simulink model "ACC_detailed_model2"  (R2018a)
settings: Solver=VariableStepAuto  StartTime=0.0  StopTime=250  FixedStep=1e-3  RelTol=1e-3
InitFcn:
  | Jw = 4.5; % Inertia Kg.m^2
  | r = 0.3; % Radius of Wheel
  | Cf = 0.1; % Viscous coefficient
  | 
  | r=0.3; % Radius of wheel
  |  %Dry Asphalt road%
  | C1 = 1.2801;
  | C2 = 23.99;
  | C3 = 0.52;
  | 
  | M = 1300; % 1500Kg
  | g = 9.81; % m/s2
  | Cr = 0.01;				% coefficient of rolling friction
  | rho = 1.3;				% density of air, kg/m^3
  | Cd = 0.46;% drag coefficient
  | 
  | maxspeed=30;
  | Alarm1=0;  %Initializing the Alarm
  | speed1=0;  %Initializing the speed
  | Default_Spacing_distance = 5; % Default Safe distance between both vehicles
  | THW= 1.5; %Time Headway
  | min_distance = 2; % Minimum Distance
libraries: simulink x5
settings Model: Creator=CHIZOM WORNU  LastModifiedBy=CHIZOM WORNU
settings SolverCC: ConsecutiveZCsStepRelTol=1*128*eps  ZeroCrossControl=EnableAll  ZeroCrossAlgorithm=Adaptive

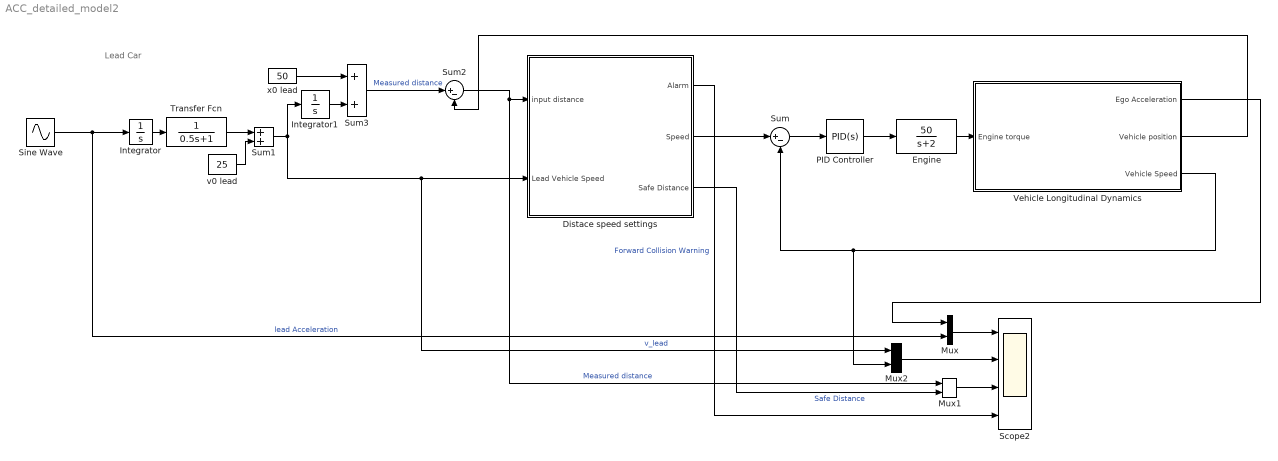
== system ACC_detailed_model2 ==
  note: Lead Car
  Distace speed settings : Subsystem
  Engine : TransferFcn  Numerator=50  Denominator=[1 2]
  Integrator : Integrator
  Integrator1 : Integrator  InitialCondition=10
  Mux : Mux  Inputs=2
  Mux1 : Mux  Inputs=2
  Mux2 : Mux  Inputs=2
  PID Controller : simulink/Continuous/PID Controller  Controller=PID  TimeDomain=Continuous-time  SampleTime=-1  IntegratorMethod=Forward Euler  FilterMethod=Forward Euler  Form=Parallel  UseFilter=on  ControllerParametersSource=internal  P=30.0096454190468  I=4.39323599940394  D=-0.171141386307986  N=175.350019457254  InitialConditionSource=internal  InitialConditionForIntegrator=0  InitialConditionForFilter=0  ExternalReset=none  LimitOutput=off  UpperSaturationLimit=inf  LowerSaturationLimit=-inf  LinearizeAsGain=on  AntiWindupMode=none  Kb=1  TrackingMode=off  Kt=1  PParamMin=[]  PParamMax=[]  IParamMin=[]  IParamMax=[]  DParamMin=[]  DParamMax=[]  NParamMin=[]  NParamMax=[]  KbParamMin=[]  KbParamMax=[]  KtParamMin=[]  KtParamMax=[]  POutMin=[]  POutMax=[]  IOutMin=[]  IOutMax=[]  DOutMin=[]  DOutMax=[]  NOutMin=[]  NOutMax=[]  KbOutMin=[]  KbOutMax=[]  KtOutMin=[]  KtOutMax=[]  IntegratorOutMin=[]  IntegratorOutMax=[]  FilterOutMin=[]  FilterOutMax=[]  SumOutMin=[]  SumOutMax=[]  SumI1OutMin=[]  SumI1OutMax=[]  SumI2OutMin=[]  SumI2OutMax=[]  SumI3OutMin=[]  SumI3OutMax=[]  SumDOutMin=[]  SumDOutMax=[]  SaturationOutMin=[]  SaturationOutMax=[]  IntegratorContinuousStateAttributes=''  IntegratorStateMustResolveToSignalObject=off  IntegratorRTWStateStorageClass=Auto  FilterContinuousStateAttributes=''  FilterStateMustResolveToSignalObject=off  FilterRTWStateStorageClass=Auto  DifferentiatorICPrevScaledInput=0  DifferentiatorOutMin=[]  DifferentiatorOutMax=[]  InitialConditionSetting=State (most efficient)  FilterDiffOutCoefMin=[]  FilterDiffOutCoefMax=[]  SumDenOutMin=[]  SumDenOutMax=[]  SumNumOutMin=[]  SumNumOutMax=[]  ReciprocalOutMin=[]  ReciprocalOutMax=[]  DivideOutMin=[]  DivideOutMax=[]  TunerSelectOption=Transfer Function Based (PID Tuner App)
  Scope2 : Scope  NumInputPorts=4
  Sine Wave : Sin  Amplitude=0.5  Frequency=0.2  SampleTime=0.1
  Sum : Sum  Inputs=|+-
  Sum1 : Sum
  Sum2 : Sum  Inputs=|+-
  Sum3 : Sum
  Transfer Fcn : TransferFcn  Denominator=[0.5 1]
  Vehicle Longitudinal Dynamics : Subsystem
  v0 lead : Constant  Value=25  SampleTime=0.1
  x0 lead : Constant  Value=50  SampleTime=0.1
  wires:
  Mux/1 -> Scope2/1
  Sum/1 -> PID Controller/1
  PID Controller/1 -> Engine/1
  Sum2/1 -> Distace speed settings/1(input distance), Mux1/1  "Measured distance"
  Sum1/1 -> Distace speed settings/2(Lead Vehicle Speed), Mux2/1, Integrator1/1  "v_lead"
  Sine Wave/1 -> Mux/2, Integrator/1  "lead Acceleration"
  Sum3/1 -> Sum2/1  "Measured distance"
  Mux2/1 -> Scope2/2
  Mux1/1 -> Scope2/3
  Integrator1/1 -> Sum3/2
  x0 lead/1 -> Sum3/1
  Integrator/1 -> Transfer Fcn/1
  v0 lead/1 -> Sum1/2
  Transfer Fcn/1 -> Sum1/1
  Engine/1 -> Vehicle Longitudinal Dynamics/1(Engine torque)
  Vehicle Longitudinal Dynamics/1(Ego Acceleration) -> Mux/1
  Distace speed settings/1(Alarm) -> Scope2/4  "Forward Collision Warning"
  Distace speed settings/2(Speed) -> Sum/1
  Distace speed settings/3(Safe Distance) -> Mux1/2  "Safe Distance"
  Vehicle Longitudinal Dynamics/2(Vehicle position) -> Sum2/2
  Vehicle Longitudinal Dynamics/3(Vehicle Speed) -> Sum/2, Mux2/2

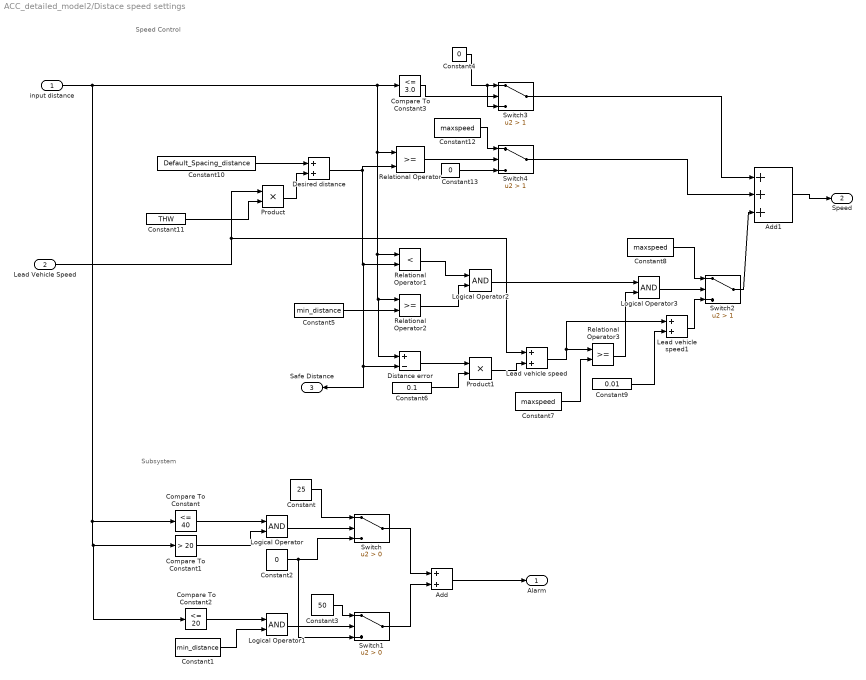
== system ACC_detailed_model2/Distace speed settings ==
  note: Speed Control
  note: Subsystem
  input distance : Inport
  Lead Vehicle Speed : Inport  Port=2
  Add : Sum
  Add1 : Sum  Inputs=3
  Compare To Constant : simulink/Logic and Bit Operations/Compare To Constant  relop=<=  const=40  OutDataTypeStr=boolean
  Compare To Constant1 : simulink/Logic and Bit Operations/Compare To Constant  relop=>  const=20  OutDataTypeStr=boolean
  Compare To Constant2 : simulink/Logic and Bit Operations/Compare To Constant  relop=<=  const=20  OutDataTypeStr=boolean
  Compare To Constant3 : simulink/Logic and Bit Operations/Compare To Constant  relop=<=  const=3.0  OutDataTypeStr=boolean
  Constant : Constant  Value=25
  Constant1 : Constant  Value=min_distance
  Constant10 : Constant  Value=Default_Spacing_distance
  Constant11 : Constant  Value=THW
  Constant12 : Constant  Value=maxspeed
  Constant13 : Constant  Value=0
  Constant2 : Constant  Value=0
  Constant3 : Constant  Value=50
  Constant4 : Constant  Value=0
  Constant5 : Constant  Value=min_distance
  Constant6 : Constant  Value=0.1
  Constant7 : Constant  Value=maxspeed
  Constant8 : Constant  Value=maxspeed
  Constant9 : Constant  Value=0.01
  Desired distance : Sum
  Distance error : Sum  Inputs=+-
  Lead vehicle speed : Sum
  Lead vehicle speed1 : Sum
  Logical Operator{,1..3} (4 alike) : Logic  AllPortsSameDT=off  OutDataTypeStr=boolean
  Product : Product
  Product1 : Product
  Relational Operator : RelationalOperator  OutDataTypeStr=boolean  RndMeth=Simplest
  Relational Operator1 : RelationalOperator  Operator=<  OutDataTypeStr=boolean  RndMeth=Simplest
  Relational Operator2 : RelationalOperator  OutDataTypeStr=boolean  RndMeth=Simplest
  Relational Operator3 : RelationalOperator  OutDataTypeStr=boolean  RndMeth=Simplest
  Switch : Switch  Criteria=u2 > Threshold
  Switch1 : Switch  Criteria=u2 > Threshold
  Switch2 : Switch  Criteria=u2 > Threshold  Threshold=1
  Switch3 : Switch  Criteria=u2 > Threshold  Threshold=1
  Switch4 : Switch  Criteria=u2 > Threshold  Threshold=1
  Alarm : Outport
  Speed : Outport  Port=2
  Safe Distance : Outport  Port=3
  wires:
  Add/1 -> Alarm/1
  Lead vehicle speed/1 -> Lead vehicle speed1/1, Relational Operator3/1
  Add1/1 -> Speed/1
  Desired distance/1 -> Distance error/2, Safe Distance/1, Relational Operator1/2, Relational Operator/2
  Switch/1 -> Add/1
  Constant1/1 -> Logical Operator1/2
  Constant3/1 -> Switch1/1
  Logical Operator1/1 -> Switch1/2
  Compare To Constant/1 -> Logical Operator/1
  Logical Operator/1 -> Switch/2
  Compare To Constant1/1 -> Logical Operator/2
  Constant2/1 -> Switch1/3, Switch/3
  Switch1/1 -> Add/2
  Constant/1 -> Switch/1
  Compare To Constant2/1 -> Logical Operator1/1
  Switch3/1 -> Add1/1
  Constant13/1 -> Switch4/3
  Constant10/1 -> Desired distance/1
  Constant9/1 -> Lead vehicle speed1/2
  Constant4/1 -> Switch3/3, Switch3/1
  Product1/1 -> Lead vehicle speed/2
  Relational Operator1/1 -> Logical Operator2/1
  Constant8/1 -> Switch2/1
  Lead vehicle speed1/1 -> Switch2/3
  Distance error/1 -> Product1/1
  Constant5/1 -> Relational Operator2/2
  Relational Operator/1 -> Switch4/2
  Product/1 -> Desired distance/2
  Constant11/1 -> Product/2
  Constant7/1 -> Relational Operator3/2
  Switch2/1 -> Add1/3
  Constant12/1 -> Switch4/1
  Logical Operator2/1 -> Logical Operator3/1
  Switch4/1 -> Add1/2
  Logical Operator3/1 -> Switch2/2
  Constant6/1 -> Product1/2
  Compare To Constant3/1 -> Switch3/2
  Lead Vehicle Speed/1 -> Product/1, Lead vehicle speed/1
  Relational Operator3/1 -> Logical Operator3/2
  input distance/1 -> Compare To Constant2/1, Compare To Constant1/1, Compare To Constant/1, Compare To Constant3/1, Distance error/1, Relational Operator2/1, Relational Operator1/1, Relational Operator/1
  Relational Operator2/1 -> Logical Operator2/2

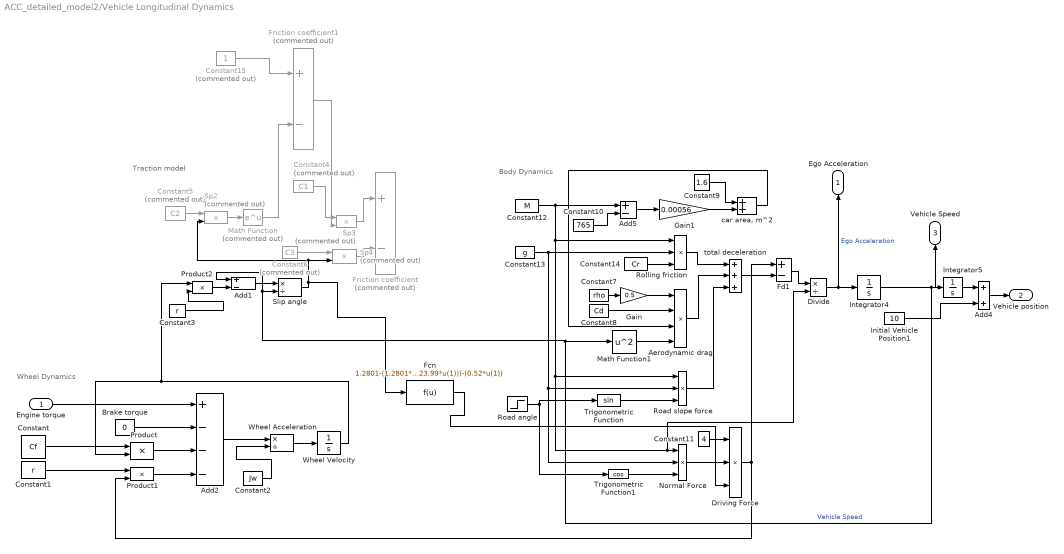
== system ACC_detailed_model2/Vehicle Longitudinal Dynamics ==
  note: Body Dynamics
  note: Traction model
  note: Wheel Dynamics
  Engine torque : Inport
  Add1 : Sum  Inputs=+-
  Add2 : Sum  Inputs=+---
  Add4 : Sum
  Add5 : Sum  Inputs=+-
  Aerodynamic drag : Product  Inputs=4
  Brake torque : Constant  Value=0
  Constant : Constant  Value=Cf
  Constant1 : Constant  Value=r
  Constant10 : Constant  Value=765
  Constant11 : Constant  Value=4
  Constant12 : Constant  Value=M
  Constant13 : Constant  Value=g
  Constant14 : Constant  Value=Cr
  Constant15 : Constant  Commented=on
  Constant2 : Constant  Value=Jw
  Constant3 : Constant  Value=r
  Constant4 : Constant  Commented=on  Value=C1
  Constant5 : Constant  Commented=on  Value=C2
  Constant6 : Constant  Commented=on  Value=C3
  Constant7 : Constant  Value=rho
  Constant8 : Constant  Value=Cd
  Constant9 : Constant  Value=1.6
  Divide : Product  Inputs=*/
  Driving Force : Product  Inputs=3
  Fcn : Fcn  Expr=1.2801-(1.2801*exp(23.99*u(1)))-(0.52*u(1))
  Fd1 : Sum  Inputs=+-
  Friction coefficient : Sum  Commented=on  Inputs=+-
  Friction coefficient1 : Sum  Commented=on  Inputs=+-
  Gain : Gain  Gain=0.5
  Gain1 : Gain  Gain=0.00056
  Initial Vehicle Position1 : Constant  Value=10  SampleTime=0.1
  Integrator4 : Integrator  InitialCondition=1
  Integrator5 : Integrator  InitialCondition=1
  Math Function : Math  Commented=on  SaturateOnIntegerOverflow=on
  Math Function1 : Math  Operator=square  SaturateOnIntegerOverflow=on
  Normal Force : Product  Inputs=3
  Product : Product
  Product1 : Product
  Product2 : Product
  Road angle : Step  Time=50  After=0  SampleTime=0
  Road slope force : Product  Inputs=3
  Rolling friction : Product  Inputs=3
  Slip angle : Product  Inputs=*/
  Sp2 : Product  Commented=on  Inputs=**
  Sp3 : Product  Commented=on  Inputs=**
  Sp4 : Product  Commented=on  Inputs=**
  Trigonometric Function : Trigonometry
  Trigonometric Function1 : Trigonometry  Operator=cos
  Wheel Acceleration : Product  Inputs=*/
  Wheel Velocity : Integrator
  "car area, m^2" : Sum
  total deceleration : Sum  Inputs=3
  Ego Acceleration : Outport
  Vehicle position : Outport  Port=2
  Vehicle Speed : Outport  Port=3
  wires:
  Divide/1 -> Ego Acceleration/1, Integrator4/1  "Ego Acceleration"
  Constant13/1 -> Normal Force/2, Road slope force/2, Rolling friction/2
  Wheel Velocity/1 -> Product/2, Product2/1
  Constant12/1 -> Divide/2, Normal Force/1, Road slope force/1, Rolling friction/1, Add5/1
  Wheel Acceleration/1 -> Wheel Velocity/1
  total deceleration/1 -> Fd1/2
  Trigonometric Function/1 -> Road slope force/3
  Add2/1 -> Wheel Acceleration/1
  Trigonometric Function1/1 -> Normal Force/3
  "car area, m^2"/1 -> Aerodynamic drag/3
  Constant1/1 -> Product1/1
  Driving Force/1 -> Fd1/1, Product1/2
  Product/1 -> Add2/3
  Math Function/1 -> Friction coefficient1/2
  Constant/1 -> Product/1
  Integrator4/1 -> Vehicle Speed/1, Integrator5/1, Math Function1/1, Slip angle/2, Add1/1  "Vehicle Speed"
  Product1/1 -> Add2/4
  Normal Force/1 -> Driving Force/2
  Road slope force/1 -> total deceleration/3
  Gain1/1 -> "car area, m^2"/2
  Constant2/1 -> Wheel Acceleration/2
  Brake torque/1 -> Add2/2
  Slip angle/1 -> Fcn/1, Sp4/2, Sp2/2
  Aerodynamic drag/1 -> total deceleration/2
  Constant4/1 -> Sp3/1
  Sp3/1 -> Friction coefficient/1
  Fd1/1 -> Divide/1
  Road angle/1 -> Trigonometric Function/1, Trigonometric Function1/1
  Constant7/1 -> Gain/1
  Sp4/1 -> Friction coefficient/2
  Constant5/1 -> Sp2/1
  Add1/1 -> Slip angle/1
  Constant14/1 -> Rolling friction/3
  Sp2/1 -> Math Function/1
  Constant10/1 -> Add5/2
  Gain/1 -> Aerodynamic drag/1
  Constant3/1 -> Product2/2
  Constant6/1 -> Sp4/1
  Constant11/1 -> Driving Force/1
  Product2/1 -> Add1/2
  Constant9/1 -> "car area, m^2"/1
  Fcn/1 -> Driving Force/3
  Rolling friction/1 -> total deceleration/1
  Initial Vehicle Position1/1 -> Add4/2
  Integrator5/1 -> Add4/1
  Add5/1 -> Gain1/1
  Constant8/1 -> Aerodynamic drag/2
  Engine torque/1 -> Add2/1
  Add4/1 -> Vehicle position/1
  Math Function1/1 -> Aerodynamic drag/4
  Constant15/1 -> Friction coefficient1/1
  Friction coefficient1/1 -> Sp3/2
